simulink model "cw6_model_BORKOWSKI"  (R2024a)
settings: Solver=VariableStepAuto  StartTime=0.0  StopTime=300  MaxStep=0.01  MinStep=0.001  RelTol=1e-6
values from neighbouring files (symbols this model uses):
  A = [-a0 a0; a1 -a1-a2]    [cw6_dane_BORKOWSKI.m]
  a0 = 1/(R1 *C1)    (= 0.1)    [cw6_dane_BORKOWSKI.m]
  a1 = 1/(R1*C2)    (= 0.2)    [cw6_dane_BORKOWSKI.m]
  a2 = 1/(R2*C2)    (= 0.1)    [cw6_dane_BORKOWSKI.m]
  B = [b1; 0]    [cw6_dane_BORKOWSKI.m]
  b1 = 1/C1    (= 0.1)    [cw6_dane_BORKOWSKI.m]
  C = [0 1]    [cw6_dane_BORKOWSKI.m]
  D = [0]    [cw6_dane_BORKOWSKI.m]
settings Model: Creator=Student  LastModifiedBy=Kamil
settings SolverCC: AlgebraicLoopSolver=TrustRegion
settings DataIOCC: SaveFormat=Array  ReturnWorkspaceOutputs=off
settings DebuggingCC: ArithmeticOperatorsInVariantConditions=warning
settings SFSimCC: CustomCodeUndefinedFunction=UseInterfaceOnly
settings RTWCC: GPUComputeCapability=3.5

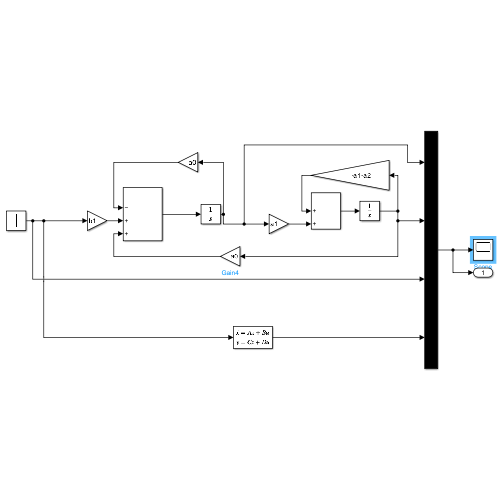
[thumbnail: Simulink's stored preview of the top-level diagram]
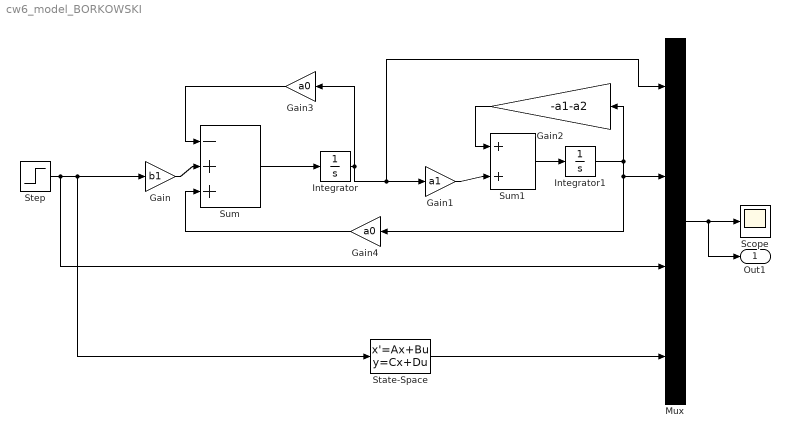
== system cw6_model_BORKOWSKI ==
  Gain : Gain  Gain=b1
  Gain1 : Gain  Gain=a1
  Gain2 : Gain  Gain=-a1-a2
  Gain3 : Gain  Gain=a0
  Gain4 : Gain  Gain=a0
  Integrator : Integrator
  Integrator1 : Integrator
  Mux : Mux
  Scope : Scope
  State-Space : StateSpace  A=A  B=B  C=C  D=D  InitialCondition=0
  Step : Step  Time=0  SampleTime=0
  Sum : Sum  Inputs=|-++
  Sum1 : Sum  Inputs=|++
  Out1 : Outport
  wires:
  Step/1 -> Mux/3, State-Space/1, Gain/1
  Integrator/1 -> Mux/1, Gain1/1, Gain3/1
  Gain/1 -> Sum/2
  Sum/1 -> Integrator/1
  Gain1/1 -> Sum1/2
  Gain3/1 -> Sum/1
  Sum1/1 -> Integrator1/1
  Integrator1/1 -> Gain4/1, Mux/2, Gain2/1
  Gain2/1 -> Sum1/1
  Mux/1 -> Scope/1, Out1/1
  State-Space/1 -> Mux/4
  Gain4/1 -> Sum/3
